simulink model "ampli_simu"  (R2022a)
settings: Solver=VariableStepAuto  StartTime=0.0  StopTime=0.003  RelTol=1e-3
values from neighbouring files (symbols this model uses):
  C1 = 0.1e-6    (= 1e-07)    [Amplificador_operacional.m]    (also in Parametros_AO.m)
  C2 = C1    (= 1e-07)    [Amplificador_operacional.m]    (also in Parametros_AO.m)
  R1 = 1e3    (= 1000)    [Amplificador_operacional.m]    (also in Parametros_AO.m)
  R2 = R1    (= 1000)    [Amplificador_operacional.m]    (also in Parametros_AO.m)
  R3 = 10e3    (= 10000)    [Amplificador_operacional.m]    (also in Parametros_AO.m)
  R4 = 15e3    (= 15000)    [Amplificador_operacional.m]    (also in Parametros_AO.m)
  VIN = 1    [Amplificador_operacional.m]    (also in Parametros_AO.m)
settings Model: Creator=ivsid  LastModifiedBy=ivsid

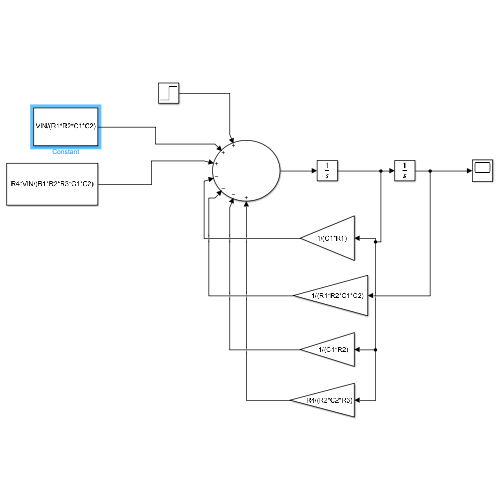
[thumbnail: Simulink's stored preview of the top-level diagram]
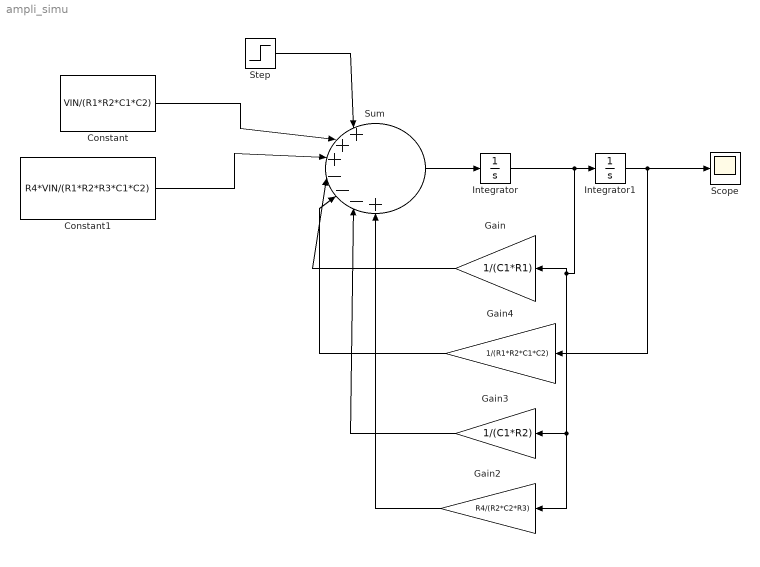
== system ampli_simu ==
  Constant : Constant  Value=VIN/(R1*R2*C1*C2)
  Constant1 : Constant  Value=R4*VIN/(R1*R2*R3*C1*C2)
  Gain : Gain  Gain=1/(C1*R1)
  Gain2 : Gain  Gain=R4/(R2*C2*R3)
  Gain3 : Gain  Gain=1/(C1*R2)
  Gain4 : Gain  Gain=1/(R1*R2*C1*C2)
  Integrator : Integrator
  Integrator1 : Integrator
  Scope : Scope
  Step : Step  SampleTime=0
  Sum : Sum  Inputs=|+++---+
  wires:
  Sum/1 -> Integrator/1
  Integrator/1 -> Gain2/1, Gain3/1, Gain/1, Integrator1/1
  Integrator1/1 -> Gain4/1, Scope/1
  Gain/1 -> Sum/4
  Gain4/1 -> Sum/5
  Gain3/1 -> Sum/6
  Gain2/1 -> Sum/7
  Step/1 -> Sum/1
  Constant/1 -> Sum/2
  Constant1/1 -> Sum/3
